simulink model "modelfit"  (R2017b)
settings: Solver=VariableStepAuto  StartTime=0.0  StopTime=10.0  RelTol=1e-3
undefined symbols (not defined in the file or in its folder): A, bf, br, cd, g, hcog, J, l, lf, lr, m, rho
settings Model: Creator=chitr  LastModifiedBy=chitr

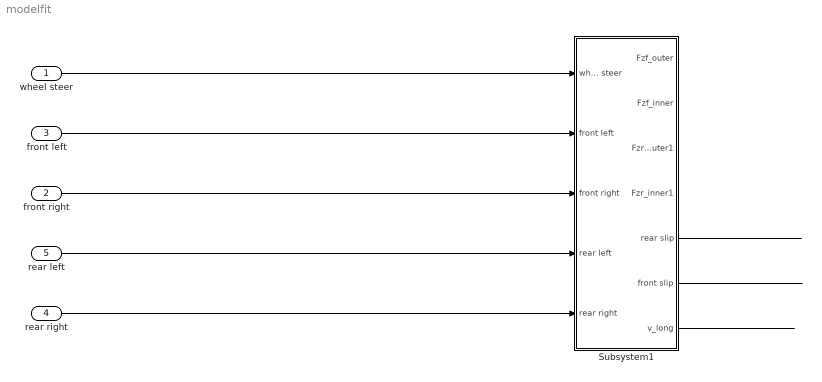
== system modelfit ==
  wheel steer : Inport
  front right : Inport  Port=2
  front left : Inport  Port=3
  rear right : Inport  Port=4
  rear left : Inport  Port=5
  Subsystem1 : Subsystem
  wires:
  wheel steer/1 -> Subsystem1/1(wheel steer)
  front left/1 -> Subsystem1/2(front left)
  front right/1 -> Subsystem1/3(front right)
  rear left/1 -> Subsystem1/4(rear left)
  rear right/1 -> Subsystem1/5(rear right)
  Subsystem1/7(v_long) -> ?
  Subsystem1/6(front slip) -> ?
  Subsystem1/5(rear slip) -> ?

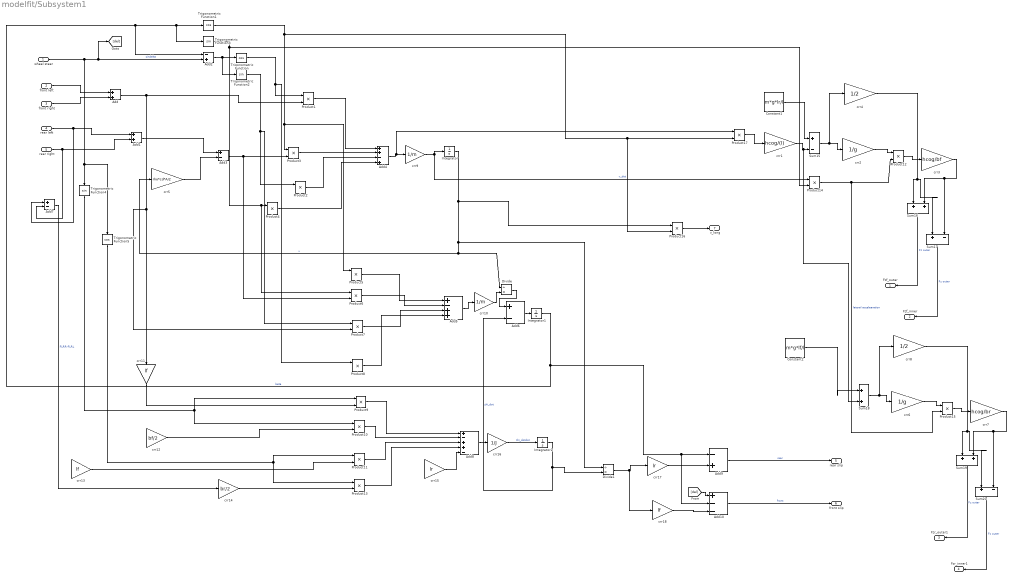
== system modelfit/Subsystem1 ==
  wheel steer : Inport
  front left : Inport  Port=2
  front right : Inport  Port=3
  rear left : Inport  Port=4
  rear right : Inport  Port=5
  Add : Sum
  Add1 : Sum
  Add10 : Sum  Inputs=+--
  Add2 : Sum  Inputs=-+
  Add3 : Sum  Inputs=+-
  Add4 : Sum  Inputs=++-+
  Add5 : Sum  Inputs=+-++
  Add6 : Sum  Inputs=+-
  Add7 : Sum  Inputs=+-
  Add8 : Sum  Inputs=+-++-
  Add9 : Sum  Inputs=-+
  Constant1 : Constant  Value=m*g*lr/l
  Constant2 : Constant  Value=m*g*lf/l
  Divide : Product  Inputs=/*
  Divide1 : Product  Inputs=/*
  Integrator : Integrator
  Integrator1 : Integrator
  Integrator2 : Integrator
  Product{1..17} (17 alike) : Product
  Sum15 : Sum  Inputs=|+-
  Sum16 : Sum  Inputs=|++
  Sum17 : Sum  Inputs=|+-
  Sum18 : Sum  Inputs=|++
  Sum19 : Sum  Inputs=|++
  Sum20 : Sum  Inputs=|+-
  Trigonometric Function : Trigonometry  Operator=cos
  Trigonometric Function1 : Trigonometry  Operator=cos
  Trigonometric Function2 : Trigonometry
  Trigonometric Function3 : Trigonometry
  Trigonometric Function4 : Trigonometry
  Trigonometric Function5 : Trigonometry  Operator=cos
  crr1 : Gain  Gain=hcog/(l)
  crr10 : Gain  Gain=1/m
  crr11 : Gain  Gain=lf
  crr12 : Gain  Gain=bf/2
  crr13 : Gain  Gain=lf
  crr14 : Gain  Gain=br/2
  crr15 : Gain  Gain=lr
  crr16 : Gain  Gain=1/J
  crr17 : Gain  Gain=lr
  crr18 : Gain  Gain=lf
  crr2 : Gain  Gain=1/g
  crr3 : Gain  Gain=hcog/bf
  crr4 : Gain  Gain=1/2
  crr5 : Gain  Gain=rho*cd*A/2
  crr6 : Gain  Gain=1/g
  crr7 : Gain  Gain=hcog/br
  crr8 : Gain  Gain=1/2
  crr9 : Gain  Gain=1/m
  "  Fzf_outer" : Outport
  Fzf_inner : Outport  Port=2
  Fzr_outer1 : Outport  Port=3
  Fzr_inner1 : Outport  Port=4
  rear slip : Outport  Port=5
  front slip : Outport  Port=6
  v_long : Outport  Port=7
  wires:
  Sum15/1 -> crr4/1, crr2/1
  crr2/1 -> Product12/1
  Product14/1 -> Product12/2, Product15/2  "lateral accelearation"
  Product12/1 -> crr3/1
  crr3/1 -> Sum17/2, Sum16/2
  crr4/1 -> Sum17/1, Sum16/1
  Sum16/1 -> "  Fzf_outer"/1  "Fz outer"
  Sum17/1 -> Fzf_inner/1  "Fz outer"
  crr6/1 -> Product15/1
  Sum20/1 -> Fzr_inner1/1  "Fz outer"
  Sum18/1 -> crr8/1, crr6/1
  Sum19/1 -> Fzr_outer1/1  "Fz outer"
  Constant2/1 -> Sum18/1
  crr7/1 -> Sum20/2, Sum19/2
  Product15/1 -> crr7/1
  crr8/1 -> Sum20/1, Sum19/1
  front left/1 -> Add/1
  front right/1 -> Add/2
  rear right/1 -> Add7/2, Add1/2
  rear left/1 -> Add7/1, Add1/1
  Add/1 -> crr11/1, Product7/2, Product1/2
  Add2/1 -> Trigonometric Function2/1, Trigonometric Function/1
  Add1/1 -> Add3/1
  crr5/1 -> Add3/2
  Product1/1 -> Add4/1
  Trigonometric Function/1 -> Product8/1, Product1/1
  Trigonometric Function1/1 -> Product16/2, Product17/2, Product5/1, Product3/1
  Trigonometric Function3/1 -> Product14/2, Product6/1, Product4/1
  Product4/1 -> Add4/4
  Product2/1 -> Add4/3
  Product3/1 -> Add4/2
  Add4/1 -> Product17/1, crr9/1
  crr9/1 -> Integrator/1, Product14/1  "v_dot"
  Integrator/1 -> Product16/1, Divide1/1, Divide/1, crr5/1  "v"
  ? -> Product5/2, Product4/2  "slip rear"
  ? -> Product8/2, Product2/2  "slip front"
  Add3/1 -> Product6/2, Product3/2
  Trigonometric Function2/1 -> Product7/1, Product2/1
  Product5/1 -> Add5/1
  Product6/1 -> Add5/2
  Product7/1 -> Add5/3
  Product8/1 -> Add5/4
  Add5/1 -> crr10/1
  crr10/1 -> Divide/2
  Divide/1 -> Add6/1
  Add6/1 -> Integrator1/1
  Integrator1/1 -> Add10/2, Add9/1, Add2/1, Trigonometric Function3/1, Trigonometric Function1/1  "beta"
  wheel steer/1 -> [del], Add2/2, Trigonometric Function5/1, Trigonometric Function4/1  "sindelta"
  Trigonometric Function4/1 -> Product10/1, Product9/1
  Trigonometric Function5/1 -> Product13/1, Product11/1
  crr11/1 -> Product9/2
  crr12/1 -> Product10/2
  ? -> crr12/1  "(cfr-cfl)*slip front"
  crr13/1 -> Product11/2
  ? -> crr13/1  "(cfr+cfl)*slip front"
  Add7/1 -> crr14/1  "FLRR-FLRL"
  crr14/1 -> Product13/2
  Product9/1 -> Add8/1
  Product10/1 -> Add8/2
  Product11/1 -> Add8/3
  Product13/1 -> Add8/4
  crr15/1 -> Add8/5
  Add8/1 -> crr16/1
  ? -> crr15/1  "rear slip"
  crr16/1 -> Integrator2/1  "zhi_dotdot"
  Integrator2/1 -> Divide1/2, Add6/2  "zhi_dot"
  Product17/1 -> crr1/1
  Constant1/1 -> Sum15/1
  crr1/1 -> Sum18/2, Sum15/2
  Divide1/1 -> crr18/1, crr17/1
  crr17/1 -> Add9/2
  crr18/1 -> Add10/3
  [del] -> Add10/1
  Add10/1 -> front slip/1  "front"
  Add9/1 -> rear slip/1  "rear"
  Product16/1 -> v_long/1
